simulink model "balancing_bot"  (R2020a)
settings: Solver=FixedStepDiscrete  StartTime=0.0  StopTime=inf  FixedStep=0.01  RelTol=1e-3  EnableMultiTasking=on
libraries: arduinolib x8, simulink x1
settings Model: SimulationMode=external  ExtModeTrigDuration=2  ExtModeArchiveFileName=data.txt  ExtModeArchiveDirName=Z:\System\Desktop\MBD_2016\Lab3\integration\data  Creator=Estra  LastModifiedBy=Alexander Grebien
settings DataIOCC: LimitDataPoints=on  ReturnWorkspaceOutputs=off
settings OptimizationCC: LifeSpan=1  MaxStackSize=64  EfficientTunableParamExpr=on
settings DebuggingCC: AllowSymbolicDim=off  SFUnexpectedBacktrackingDiag=warning  SFNoUnconditionalDefaultTransitionDiag=warning  SFExecutionAtInitializationDiag=none  ArithmeticOperatorsInVariantConditions=warning
settings HardwareCC: ProdBitPerInt=16  ProdBitPerPointer=16  ProdBitPerSizeT=16  ProdBitPerPtrDiffT=16  ProdLargestAtomicFloat=None  ProdWordSize=8  ProdHWDeviceType=Atmel->AVR
settings ModelReferenceCC: PropagateSignalLabelsOutOfModel=off
settings SFSimCC: SimUseLocalCustomCode=off  MATLABDynamicMemAlloc=off  CustomCodeUndefinedFunction=UseInterfaceOnly
settings RTWCC: SystemTargetFile=ert.tlc  HardwareBoard=Arduino Mega 2560  TemplateMakefile=ert_default_tmf  RTWUseLocalCustomCode=off  Toolchain=Arduino AVR  BuildConfiguration=Faster Runs
settings CodeAppCC: MangleLength=10  StateflowObjectComments=on
settings ERTTargetCC: MultiwordLength=2048  ERTCustomFileBanners=off  SupportContinuousTime=on  SupportNonInlinedSFcns=on  RemoveResetFunc=off  SupportVariableSizeSignals=on  ModelStepFunctionPrototypeControlCompliant=off  ConvertIfToSwitch=off  SuppressUnreachableDefaultCases=off
settings ConfigComp: CovMetricSettings=dw  CovHtmlReporting=on  CovSaveCumulativeToWorkspaceVar=on  CovSaveSingleToWorkspaceVar=on  CovExternalEMLEnable=off

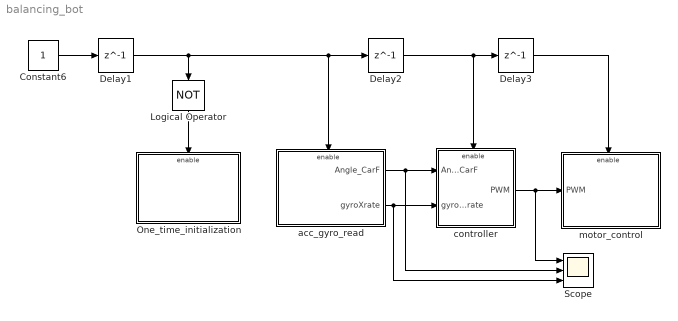
== system balancing_bot ==
  Constant6 : Constant  OutDataTypeStr=boolean  SampleTime=-1
  Delay1 : Delay  DelayLength=1
  Delay2 : Delay  DelayLength=1
  Delay3 : Delay  DelayLength=1
  Logical Operator : Logic  Operator=NOT  AllPortsSameDT=off  OutDataTypeStr=boolean
  One_time_initialization : Subsystem  TreatAsAtomicUnit=on
  Scope : Scope  NumInputPorts=3
  acc_gyro_read : Subsystem
  controller : Subsystem
  motor_control : Subsystem
  wires:
  Constant6/1 -> Delay1/1
  Logical Operator/1 -> One_time_initialization/Enable
  Delay1/1 -> acc_gyro_read/Enable, Delay2/1, Logical Operator/1
  Delay3/1 -> motor_control/Enable
  acc_gyro_read/1(Angle_CarF) -> Scope/2, controller/1(Angle_CarF)
  acc_gyro_read/2(gyroXrate) -> Scope/3, controller/2(gyroXrate)
  Delay2/1 -> controller/Enable, Delay3/1
  controller/1(PWM) -> Scope/1, motor_control/1(PWM)

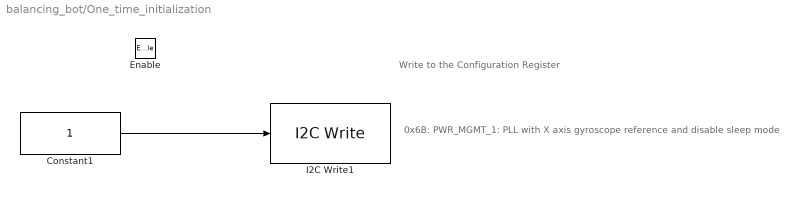
== system balancing_bot/One_time_initialization ==
  note: Write to the Configuration Register
  note: 0x6B: PWR_MGMT_1: PLL with X axis gyroscope reference and disable sleep mode
  Enable : EnablePort
  Constant1 : Constant  OutDataTypeStr=uint8  SampleTime=-1
  I2C Write1 : arduinolib/I2C Write  Priority=1  I2CModule=0  Mode=Master  SlaveAddress=hex2dec( '68' )  SlaveByteOrder=LittleEndian  Direction=Transmitter  RegisterAddressMode=on  RegisterAddress=hex2dec('6B')  SlaveDataType=uint8  DataLength=1  NoAck=off  RepeatedStart=off  OutputStatus=off  blockPlatform=arduino
      settings: AttributesFormatString=Priority=%<Priority>  SourceProductBaseCode=ARDUINO
  wires:
  Constant1/1 -> I2C Write1/1

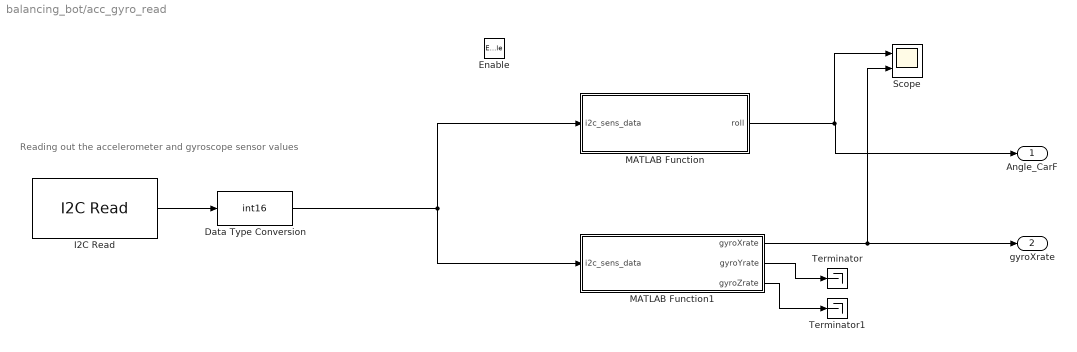
== system balancing_bot/acc_gyro_read ==
  note: Reading out the accelerometer and gyroscope sensor values
  Enable : EnablePort
  Data Type Conversion : DataTypeConversion  OutDataTypeStr=int16
  I2C Read : arduinolib/I2C Read  Priority=3  I2CModule=0  Mode=Master  SlaveAddress=hex2dec( '68' )  SlaveByteOrder=BigEndian  Direction=Receiver  RegisterAddressMode=on  RegisterAddress=hex2dec( '3B' )  SlaveDataType=uint16  DataLength=7  NoAck=off  RepeatedStart=off  OutputStatus=off  blockPlatform=arduino  SampleTime=-1
      settings: SourceProductBaseCode=ARDUINO
  MATLAB Function : MATLAB Function  TreatAsAtomicUnit=on
  MATLAB Function1 : MATLAB Function  TreatAsAtomicUnit=on
  Scope : Scope  NumInputPorts=2
  Terminator : Terminator
  Terminator1 : Terminator
  Angle_CarF : Outport  VectorParamsAs1DForOutWhenUnconnected=off
  gyroXrate : Outport  Port=2  VectorParamsAs1DForOutWhenUnconnected=off
  wires:
  I2C Read/1 -> Data Type Conversion/1
  MATLAB Function/1(roll) -> Scope/1, Angle_CarF/1
  MATLAB Function1/1(gyroXrate) -> Scope/2, gyroXrate/1
  MATLAB Function1/2(gyroYrate) -> Terminator/1
  MATLAB Function1/3(gyroZrate) -> Terminator1/1
  Data Type Conversion/1 -> MATLAB Function/1(i2c_sens_data), MATLAB Function1/1(i2c_sens_data)

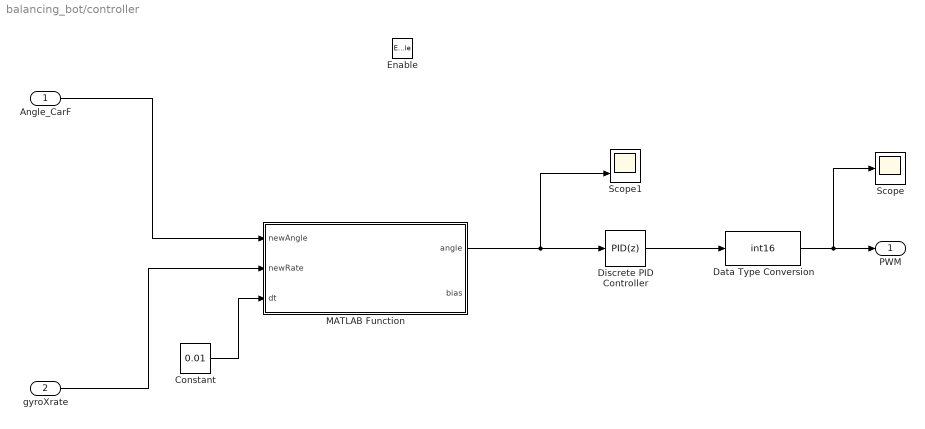
== system balancing_bot/controller ==
  Angle_CarF : Inport
  gyroXrate : Inport  Port=2
  Enable : EnablePort
  Constant : Constant  Value=0.01
  Data Type Conversion : DataTypeConversion  OutDataTypeStr=int16
  Discrete PID Controller : simulink/Continuous/PID Controller  Controller=PID  Form=Ideal  TimeDomain=Discrete-time  UseExternalTs=off  SampleTime=-1  IntegratorMethod=Forward Euler  FilterMethod=Forward Euler  ControllerParametersSource=internal  P=6  I=5  D=0.5  UseFilter=off  N=800  TunerSelectOption=Frequency Response Based  InitialConditionSource=internal  InitialConditionForIntegrator=0  InitialConditionForFilter=0  DifferentiatorICPrevScaledInput=0  ExternalReset=none  TrackingMode=off  Kt=1  LimitOutput=on  UpperSaturationLimit=255  LowerSaturationLimit=-255  LinearizeAsGain=off  AntiWindupMode=clamping  Kb=1  POutMin=[]  POutMax=[]  IOutMin=[]  IOutMax=[]  DOutMin=[]  DOutMax=[]  NOutMin=[]  NOutMax=[]  SumOutMin=[]  SumOutMax=[]  SaturationOutMin=[]  SaturationOutMax=[]  PParamMin=[]  PParamMax=[]  IParamMin=[]  IParamMax=[]  DParamMin=[]  DParamMax=[]  NParamMin=[]  NParamMax=[]  KbParamMin=[]  KbParamMax=[]  KtParamMin=[]  KtParamMax=[]  KbOutMin=[]  KbOutMax=[]  KtOutMin=[]  KtOutMax=[]  IntegratorOutMin=[]  IntegratorOutMax=[]  FilterOutMin=[]  FilterOutMax=[]  SumI1OutMin=[]  SumI1OutMax=[]  SumI2OutMin=[]  SumI2OutMax=[]  SumI3OutMin=[]  SumI3OutMax=[]  SumI4OutMin=[]  SumI4OutMax=[]  SumDOutMin=[]  SumDOutMax=[]  DifferentiatorOutMin=[]  DifferentiatorOutMax=[]  FilterDiffOutCoefMin=[]  FilterDiffOutCoefMax=[]  ReciprocalOutMin=[]  ReciprocalOutMax=[]  SumDenOutMin=[]  SumDenOutMax=[]  SumNumOutMin=[]  SumNumOutMax=[]  DivideOutMin=[]  DivideOutMax=[]  UdiffTsProdOutMin=[]  UdiffTsProdOutMax=[]  NTsProdOutMin=[]  NTsProdOutMax=[]  UintegralTsProdOutMin=[]  UintegralTsProdOutMax=[]  UngainTsProdOutMin=[]  UngainTsProdOutMax=[]  IntegratorContinuousStateAttributes=''  IntegratorStateMustResolveToSignalObject=off  IntegratorRTWStateStorageClass=Auto  FilterContinuousStateAttributes=''  FilterStateMustResolveToSignalObject=off  FilterRTWStateStorageClass=Auto  ParallelPVariant=Passthrough  IdealPVariant=InternalParameters  IVariant=InternalParameters  DVariant=InternalParameters  IntegratorVariant=Discrete  SatVariant=Enabled  AWVariant=DiscClampingIdeal  PCopyVariant=InternalParamsIdeal  TRVariant=Disabled  FdbkBlocksVariant=Forward  IdealPFdbkVariant=Disabled  SatFdbkVariant=Disabled  DerivativeFilterVariant=Differentiator  NVariant=Passthrough  NCopyVariant=Disabled_SignalSpec  FilterICVariant=InternalICsDifferentiator  IntegratorICVariant=InternalICs  ExternalResetVariant=Disabled  TRSumVariant=Passthrough  SumFdbkVariant=Disabled  SumVariant=Sum_PID  TsampFilterVariant=InternalTs  TsampNgainVariant=Passthrough  TsampIntegralVariant=Passthrough
  MATLAB Function : MATLAB Function  TreatAsAtomicUnit=on
  Scope : Scope
  Scope1 : Scope  NumInputPorts=2
  PWM : Outport  VectorParamsAs1DForOutWhenUnconnected=off
  wires:
  Discrete PID Controller/1 -> Data Type Conversion/1
  Angle_CarF/1 -> MATLAB Function/1(newAngle)
  gyroXrate/1 -> MATLAB Function/2(newRate)
  MATLAB Function/1(angle) -> Scope1/2, Discrete PID Controller/1
  Constant/1 -> MATLAB Function/3(dt)
  Data Type Conversion/1 -> Scope/1, PWM/1

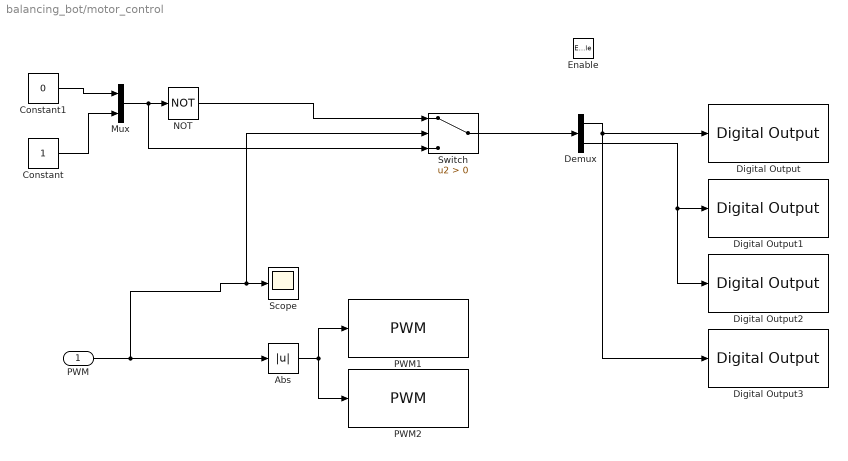
== system balancing_bot/motor_control ==
  PWM : Inport
  Enable : EnablePort
  Abs : Abs
  Constant : Constant
  Constant1 : Constant  Value=0
  Demux : Demux  Outputs=2
  Digital Output : arduinolib/Digital Output  pinNumber=8  Direction=output  blockPlatform=arduino
  Digital Output1 : arduinolib/Digital Output  pinNumber=7  Direction=output  blockPlatform=arduino
  Digital Output2 : arduinolib/Digital Output  pinNumber=3  Direction=output  blockPlatform=arduino
  Digital Output3 : arduinolib/Digital Output  pinNumber=4  Direction=output  blockPlatform=arduino
  Mux : Mux  Inputs=2
  NOT : Logic  Operator=NOT  AllPortsSameDT=off  OutDataTypeStr=boolean
  PWM1 : arduinolib/PWM  pinNumber=6  frequencyType=Default  desiredFrequency=490.2  achievableFrequency=490.2
  PWM2 : arduinolib/PWM  pinNumber=5  frequencyType=Default  desiredFrequency=490.2  achievableFrequency=490.2
  Scope : Scope
  Switch : Switch  Criteria=u2 > Threshold
  wires:
  Mux/1 -> Switch/3, NOT/1
  Constant1/1 -> Mux/1
  Constant/1 -> Mux/2
  Demux/1 -> Digital Output/1, Digital Output3/1
  Demux/2 -> Digital Output2/1, Digital Output1/1
  Abs/1 -> PWM1/1, PWM2/1
  PWM/1 -> Abs/1, Switch/2, Scope/1
  Switch/1 -> Demux/1
  NOT/1 -> Switch/1

== matlab function balancing_bot/acc_gyro_read/MATLAB Function1 ==
  data: i2c_sens_data input; gyroXrate output; gyroYrate output; gyroZrate output
function [gyroXrate,gyroYrate,gyroZrate] = fcn(i2c_sens_data)
gyroX = double(i2c_sens_data(5));
gyroY = double(i2c_sens_data(6));
gyroZ = double(i2c_sens_data(7));
gyroXrate = gyroX/131;
gyroYrate = gyroY/131;
gyroZrate = gyroZ/131; 
end

== matlab function balancing_bot/acc_gyro_read/MATLAB Function ==
  data: i2c_sens_data input; roll output
function roll = fcn(i2c_sens_data)
accX = double(i2c_sens_data(1));
accY = double(i2c_sens_data(2));
accZ = double(i2c_sens_data(3));
roll = atan(accY / sqrt(accX * accX + accZ * accZ)) * 180/pi; 
end

== matlab function balancing_bot/controller/MATLAB Function ==
  data: newAngle input; angle output; newRate input; dt input; bias output
function [angle,bias] = KalmanFil_Balanbot(newAngle,newRate,dt)
% This script was adapted for its implementation in Simulink by R. Estrada (FHJOANNEUM 2017)
% Based on KasBot V2 - Kalman filter module - http:%www.xfirm.com/?page_id=145
 % Modified by Kristian Lauszus
% More information: http:%blog.tkjelectronics.dk/2012/09/a-practical-approach-tokalman-filter-and-how-to-implement-it
 % Discrete Kalman filter time update equations - Time Update ("Predict")
 % Update xhat - Project the state ahead

 coder.extrinsic('exist');

 % Declaration of persistent in memory variables (similar to declare global
 % variables)

 persistent init0 P K x;

 % Initialization of typical sensor and noise variances
 Q_angle = 0.001;
 Q_bias = 0.003;
 R_measure = 0.03;

 % Declaration/initialization of main static matrices and vectors
 F = [1 -dt; 0 1]; % Transition matrix
 Q = [Q_angle 0; 0 Q_bias]; % Process noise covariance matrix
 B = [dt ; 0]; % Control-input model
 H = [1 0]; % Observation model

 % SETUP: Executed only the first time
 if isempty(init0)
 init0=0;
 % Declaration/initialization of main dynamic matrix and vectors
 P = [0 0;0 0]; % Error covariance matrix
 K = [0;0]; % Kalman gain vector
 x = [0;0]; % State vector
 end
 % LOOP: Implementation of Kalman filter algorithm

 % Step 1 */
 % Calculate prior state vector
 x = F * x + B * newRate;
 % Step 2 */
 % Update estimation error covariance - Project the error covariance ahead
 P = F * P * F' + Q * dt;

 % Step 3 */
 % Update estimate with measurement zk (newAngle)
 y = newAngle - H * x;
 % Step 4 */
 % Discrete Kalman filter measurement update equations - Measurement Update ("Correct")
 S = H * P * H' + R_measure;

 % Step 5 */
 % Compute the Kalman gain
 K = P * H' / S;
 % Step 6 */
 % Update state vector
 x = x + K * y;

 % Step 7 */
 % Calculate estimation error covariance - Update the error covariance
 P = (eye(2) - K * H) * P;
 % RETURN: Update the function outputs
 angle = x(1);
 bias = x(2);
 
end
